simulink model "TestSimulink_SerialBlockExample"  (R2025b)
settings: Solver=FixedStepAuto  StartTime=0.0  StopTime=inf  FixedStep=0.01  RelTol=1e-3
undefined symbols (not defined in the file or in its folder): LF
libraries: instrumentseriallib x3
settings Model: Creator=talles  LastModifiedBy=a_jax

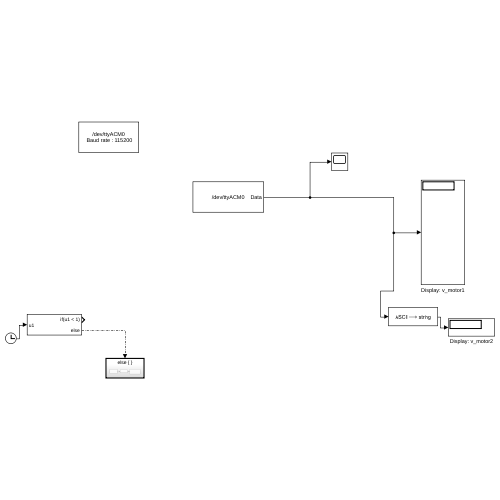
[thumbnail: Simulink's stored preview of the top-level diagram]
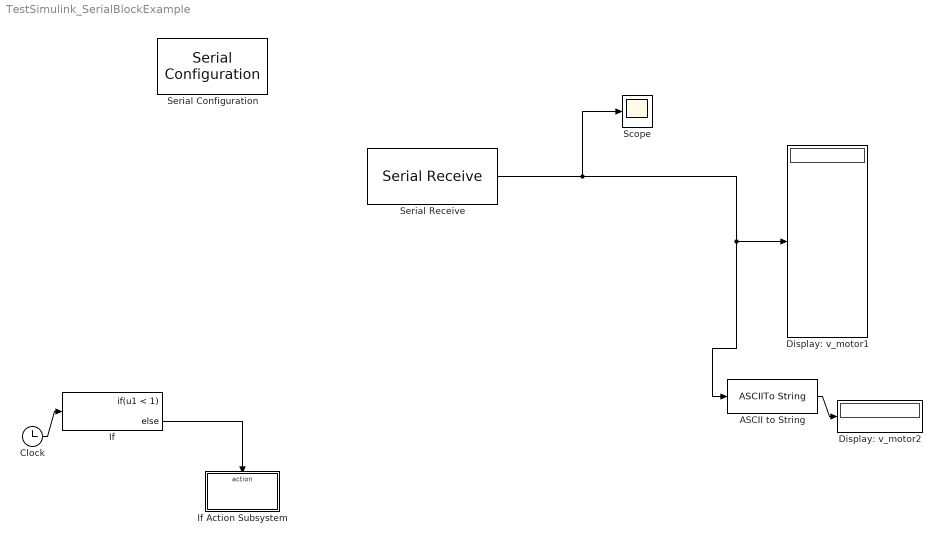
== system TestSimulink_SerialBlockExample ==
  ASCII to String : ASCIIToString
  Clock : Clock
  Display: v_motor1 : Display
      settings: Decimation=50
  Display: v_motor2 : Display
      settings: Decimation=50
  If : If  IfExpression=u1 < 1
  If Action Subsystem : Subsystem  TreatAsAtomicUnit=on
  Scope : Scope
      settings: ActiveDisplayYMinimum=4.625  ActiveDisplayYMaximum=58.375
  Serial Configuration : instrumentseriallib/Serial Configuration  Priority=-200000  PortSel=/dev/ttyACM0  Port=/dev/ttyACM0  ComPort=/dev/ttyACM0  BaudRate=115200  DataBits=8  Parity=none  StopBits=1  ByteOrder=little-endian  FlowControl=none  Timeout=0.0001  SimulateUsing=Interpreted execution  BlockInModel=on  aMode=1
      settings: LibrarySourceBlock=embeddedtargetslib/Host Communication/Serial Configuration
  Serial Receive : instrumentseriallib/Serial Receive  Priority=1  PortSel=/dev/ttyACM0  Port=/dev/ttyACM0  ComPort=/dev/ttyACM0  DataType=uint8  SaveDataType=uint8  ToggleHeader=on  Header=[10]  ToggleDataSize=on  DataSize=[10 1]  ToggleTerminator=off  Terminator=LF ('\n')  CustomTerminator=[]  InputFormat=Column major  EnableBlockingMode=on  ActionDataUnavailable=Output last received value  ActionWhenDataUnavailable=Output last received value  CustomValue=0  SampleTime=0.01  SimulateUsing=Interpreted execution  BlockInModel=on  aMode=1  LibraryInUse=instrumentlib
  wires:
  ASCII to String/1 -> Display: v_motor2/1
  Serial Receive/1 -> Scope/1, ASCII to String/1, Display: v_motor1/1
  Clock/1 -> If/1
  If/2 -> If Action Subsystem/Action

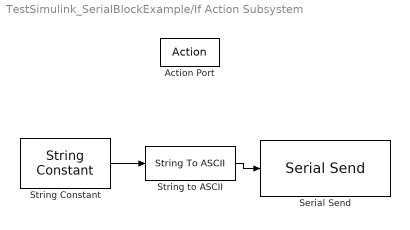
== system TestSimulink_SerialBlockExample/If Action Subsystem ==
  Action Port : ActionPort  ActionPortLabel=else
  Serial Send : instrumentseriallib/Serial Send  Priority=1  PortSel=/dev/ttyACM0  Port=/dev/ttyACM0  ComPort=/dev/ttyACM0  Header=[]  Terminator=LF ('\n')  CustomTerminator=[]  EnableBlockingMode=on  SimulateUsing=Interpreted execution  BlockInModel=on  aMode=1
  String Constant : StringConstant  String="\"1111,5556\""
  String to ASCII : StringToASCII
  wires:
  String Constant/1 -> String to ASCII/1
  String to ASCII/1 -> Serial Send/1
